simulink model "test"  (R2018b)
settings: Solver=VariableStepAuto  StartTime=0.0  StopTime=10  RelTol=1e-3
values from neighbouring files (symbols this model uses):
  A = 0.914    [KALMAN.m]    (also in main_cntl.m = eval(A_eq); main_sys.m = double(A_lin); main_sys_klm.m = double(A_lin); main_tf_0.m = A)
  b = 1    [test_1.m]
  B = 0.25    [KALMAN.m]    (also in main_cntl.m = eval(B_eq); main_sys.m = double(B_lin); main_sys_klm.m = double(B_lin); main_tf_1.m = eval(B))
  C = 0.344    [KALMAN.m]    (also in main_sys.m = double( subs( C) ); main_sys_klm.m = double( subs( C) ); main_tf_0.m = [ 0 , 0  , Ks , ds , -Ks , -ds, 0 ]; main_tf_1.m = C_mes)
  D = zeros(7,2)    [main_sys.m]    (also in main_sys_klm.m = zeros(2,2); main_tf_0.m = [ 0 , 0 ]; main_tf_1.m = zeros(1,1); main_tf_10.m = zeros(2,2))
  k = 5    [test_1.m]
  m = 10    [test_1.m]
settings Model: Creator=eshojaei  LastModifiedBy=eshojaei

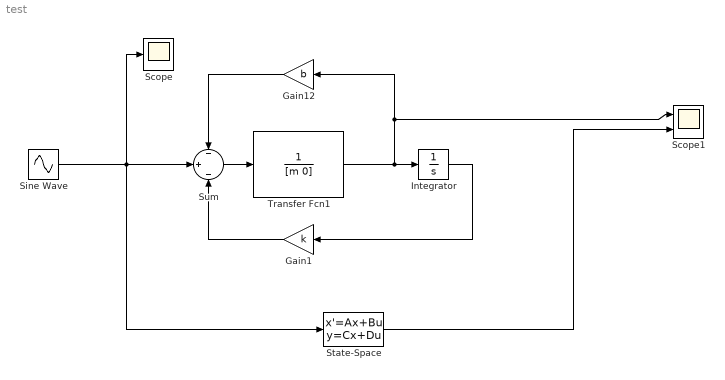
== system test ==
  Gain1 : Gain  Gain=k
  Gain12 : Gain  Gain=b
  Integrator : Integrator
  Scope : Scope
  Scope1 : Scope  NumInputPorts=2
  Sine Wave : Sin  Frequency=5  SampleTime=0
  State-Space : StateSpace  A=A  B=B  C=C  D=D  InitialCondition=0
  Sum : Sum  Inputs=-|+|-
  Transfer Fcn1 : TransferFcn  Denominator=[m 0]
  wires:
  Transfer Fcn1/1 -> Gain12/1, Scope1/1, Integrator/1
  Sine Wave/1 -> State-Space/1, Scope/1, Sum/2
  Sum/1 -> Transfer Fcn1/1
  Gain12/1 -> Sum/1
  Gain1/1 -> Sum/3
  Integrator/1 -> Gain1/1
  State-Space/1 -> Scope1/2
